simulink model "ssc_auto_ev_20b"  (R2020b)
settings: Solver=VariableStepAuto  StartTime=0.0  StopTime=200  RelTol=1e-3  AbsTol=1e-3
PreLoadFcn:
  | % Simulation parameters
  | dt = 0.01;
  | 
  | % Battery cell parameters
  | ssc_lithium_cell_1RC_ini
  | Nseries = 100;
  | Nparallel = 10;
  | 
  | % Motor parameters
  | max_torque = 220;
  | max_power = 80e3;
  | 
  | % Vehicle parameters
  | vehicle_mass = 4000;
  | wheel_radius = 0.35;
  | area = 5;
  | drag_coefficient = 0.25;
  | air_density = 1.225;
  | gravity = 9.81;
  | rolling_res_ratio = 0.015;
  | 
  | % Differential drive parameters
  | gear_ratio = 12;
  | 
  | % Simplified braking system parameters
  | force_max_pedal = 500;
  | braking_torque_to_pedal_force_ratio = -16;
  | 
  | % Vehicle controller parameters
  | hill_hold_max_speed = 0.5;
  | 
  | % Water properties for cooling circuit
  | load WaterProperties
  | 
  | % Input signals for Signal Editor block
  | load ssc_auto_ev_Inputs
values from neighbouring files (symbols this model uses):
  C1_LUT = [1913.6 4625.7 23306 10736 18036 12251 9022.9 12447 18872 40764 18721 33630 ... (21 elements, 7x3)]    [ssc_auto_ev_param.mat]
  Capacity_LUT = [28.0081 27.625 27.6392]    [ssc_auto_ev_param.mat]
  cell_Cp_heat = 810.5328    [ssc_auto_ev_param.mat]
  cell_mass = 1    [ssc_auto_ev_param.mat]
  Em_LUT = [3.4966 3.5519 3.6183 3.7066 3.9131 4.0748 4.1923 3.5057 3.566 3.6337 3.7127 3.9259 ... (21 elements, 7x3)]    [ssc_auto_ev_param.mat]
  Qe_init = 15.6845    [ssc_auto_ev_param.mat]
  R0_LUT = [0.0117 0.011 0.0114 0.0107 0.0107 0.0113 0.0116 0.0085 0.0085 0.0087 0.0082 0.0083 ... (21 elements, 7x3)]    [ssc_auto_ev_param.mat]
  R1_LUT = [0.0109 0.0069 0.0047 0.0034 0.0033 0.0033 0.0028 0.0029 0.0024 0.0026 0.0016 0.0023 ... (21 elements, 7x3)]    [ssc_auto_ev_param.mat]
  SOC_LUT = [0 0.1 0.25 0.5 0.75 0.9 1]    [ssc_auto_ev_param.mat]
  T_init = 293.15    [ssc_auto_ev_param.mat]
  Temperature_LUT = [278.15 293.15 313.15]    [ssc_auto_ev_param.mat]
undefined symbols (not defined in the file or in its folder): DiscIntNeverNeededParam, K, Lambda, tau, x0
libraries: fl_lib x656, nesl_utility x86, simulink x21, LiBatteryElements_lib x16, SignalEditorBlockLib x4, simulink_extras x4
(part 6 of 13)

== system ssc_auto_ev_20b/Step 3: Ungroup and Redraw/Motor Drive ==
  iRef : Inport
  DC Motor1 : Subsystem  Tag=PublishSubsystem
      mask Display:
      | % Circle, in/out, and 'M'
      | image('ssc_dcmotor_maskicon.png');
      | 
      | % % Circle
      | % plot(sin(0:0.1:2.2*pi)*0.9,cos(0:0.1:2.2*pi)*0.9);
      | %
      | % % In/out
      | % plot([-1.3 -0.9],[0 0]);
      | % plot([1.3 0.9],[0 0]);
      | %
      | % % 'M'
      | % plot([0.5 0.5],[-0.5 0.5]);
      | % plot([-0.5 -0.5],[-0.5 0.5]);
      | % plot([0.5 0],[0.5 -0.5]);
      | % plot([-0.5 0],[0.5 -0.5]);
      | 
      | % Plot points to set plot range
      | color('white');plot(1.5,1.5);plot(-1.5,-1.5)
      | color('black');
      | 
      | port_label('RConn',1,'R');
      | port_label('RConn',2,'C');
      | port_label('LConn',1,'V+');
      | port_label('LConn',2,'V-');
  DC Motor2 : Subsystem  Tag=PublishSubsystem
      mask Display:
      | % Circle, in/out, and 'M'
      | image('ssc_dcmotor_maskicon.png');
      | 
      | % % Circle
      | % plot(sin(0:0.1:2.2*pi)*0.9,cos(0:0.1:2.2*pi)*0.9);
      | %
      | % % In/out
      | % plot([-1.3 -0.9],[0 0]);
      | % plot([1.3 0.9],[0 0]);
      | %
      | % % 'M'
      | % plot([0.5 0.5],[-0.5 0.5]);
      | % plot([-0.5 -0.5],[-0.5 0.5]);
      | % plot([0.5 0],[0.5 -0.5]);
      | % plot([-0.5 0],[0.5 -0.5]);
      | 
      | % Plot points to set plot range
      | color('white');plot(1.5,1.5);plot(-1.5,-1.5)
      | color('black');
      | 
      | port_label('RConn',1,'R');
      | port_label('RConn',2,'C');
      | port_label('LConn',1,'V+');
      | port_label('LConn',2,'V-');
  Ideal Rotational Motion Sensor : fl_lib/Mechanical/Mechanical Sensors/Ideal Rotational Motion Sensor  wrap_angle=simscape.enum.onoff.off  offset=0 rad
      settings: SourceProductBaseCode=PW,SS,VE
  MRRef : fl_lib/Mechanical/Rotational Elements/Mechanical Rotational Reference
      settings: SourceProductBaseCode=PW,SS,VE
  MRRef1 : fl_lib/Mechanical/Rotational Elements/Mechanical Rotational Reference
      settings: SourceProductBaseCode=PW,SS,VE
  MRRef2 : fl_lib/Mechanical/Rotational Elements/Mechanical Rotational Reference
      settings: SourceProductBaseCode=PW,SS,VE
  Motor Torque Controller 1 (System-Level Representation) : Subsystem
      settings: PortSchema="{\"entries\":[{\"content\":{\"sides\":[{\"content\":{\"connectorIds\":[\"LConn1\",\"LConn2\"]},\"type\":\"ConnectorPlacement.EquallySpacedRectSide\",\"uuid\":\"fa610323-4e51-4b68-84d8-5520af174050\"},{\"content\":{\"connectorIds\":[\"RConn1\",\"RConn2\"],\"side\":\"RIGHT\"},\"type\":\"ConnectorPlacement.EquallySpacedRectSide\",\"uuid\":\"4363b90b-a4e0-4b49-9dec-cc6d130d9345\"},{\"content\":{\"connectorIds\":[\"LConn3\"],\"side\":\"TOP\"},\"type\":\"ConnectorPlacement.EquallySpacedRectSide\",\"uuid\":\"1b5285b6-bf42-4633-bccd-78a8c0464c36\"}]},\"type\":\"ConnectorPlacement.EquallySpacedConnector\",\"uuid\":\"5522e717-4ae9-420d-ac3d-a671d244aac1\"}],\"packageUris\":[\"http://schema.mathworks.com/mf0/Connector/R2020b\"],\"version\":\"1.0\"}"
  Motor Torque Controller 1 (System-Level Representation)1 : Subsystem
      settings: PortSchema="{\"entries\":[{\"content\":{\"sides\":[{\"content\":{\"connectorIds\":[\"LConn1\",\"LConn2\"]},\"type\":\"ConnectorPlacement.EquallySpacedRectSide\",\"uuid\":\"fa610323-4e51-4b68-84d8-5520af174050\"},{\"content\":{\"connectorIds\":[\"RConn1\",\"RConn2\"],\"side\":\"RIGHT\"},\"type\":\"ConnectorPlacement.EquallySpacedRectSide\",\"uuid\":\"4363b90b-a4e0-4b49-9dec-cc6d130d9345\"},{\"content\":{\"connectorIds\":[\"LConn3\"],\"side\":\"TOP\"},\"type\":\"ConnectorPlacement.EquallySpacedRectSide\",\"uuid\":\"1b5285b6-bf42-4633-bccd-78a8c0464c36\"}]},\"type\":\"ConnectorPlacement.EquallySpacedConnector\",\"uuid\":\"5522e717-4ae9-420d-ac3d-a671d244aac1\"}],\"packageUris\":[\"http://schema.mathworks.com/mf0/Connector/R2020b\"],\"version\":\"1.0\"}"
  Sensing wMotor : Subsystem
      mask Display: disp('w');
  Simulink-PS G1 : nesl_utility/Simulink-PS Converter  PhysicalDomain=network_engine_domain  SubClassName=ps_input  LeftPortType=input  RightPortType=output  PseudoPeriodic=off  Frequencies=[]  NoiseDistribution=none  NoiseParameters=[]  Unit=A  AffineConversion=off  FilteringAndDerivatives=zero  SimscapeFilterOrder=1  InputFilterTimeConstant=1e-6  UdotUserProvided=1
      settings: SourceProductBaseCode=SS,PW,VE
  Winding-Iron Conductance/1 : fl_lib/Thermal/Thermal Elements/Conductive Heat Transfer  area=250 cm^2  thickness=0.2 cm  th_cond=360 W/(m*K)  T_specify=off  T_priority=None  T=0 K  T_nominal_specify=off  T_nominal_unit=K  T_nominal_value=1  Q_specify=off  Q_priority=None  Q=0 W  Q_nominal_specify=off  Q_nominal_unit=W  Q_nominal_value=1
      settings: SourceProductBaseCode=PW,SS,VE
  Winding-Iron Conductance/2 : fl_lib/Thermal/Thermal Elements/Conductive Heat Transfer  area=250 cm^2  thickness=0.2 cm  th_cond=360 W/(m*K)  T_specify=off  T_priority=None  T=0 K  T_nominal_specify=off  T_nominal_unit=K  T_nominal_value=1  Q_specify=off  Q_priority=None  Q=0 W  Q_nominal_specify=off  Q_nominal_unit=W  Q_nominal_value=1
      settings: SourceProductBaseCode=PW,SS,VE
  + : PMIOPort  Side=Left
  - : PMIOPort  Port=2  Side=Left
  R : PMIOPort  Port=3  Side=Right
  M1 : PMIOPort  Port=4  Side=Left
  M2 : PMIOPort  Port=5  Side=Left
  w : Outport  VectorParamsAs1DForOutWhenUnconnected=off
  wires:
  iRef/1 -> Simulink-PS G1/1
  Sensing wMotor/1(SL) -> w/1
  connections:
  M2/RConn1 -- Winding-Iron Conductance/2/LConn1
  M1/RConn1 -- Winding-Iron Conductance/1/LConn1
  Winding-Iron Conductance/2/RConn1 -- DC Motor2/LConn3
  Winding-Iron Conductance/1/RConn1 -- DC Motor1/LConn3
  DC Motor2/LConn2 -- Motor Torque Controller 1 (System-Level Representation)1/LConn2
  DC Motor2/LConn1 -- Motor Torque Controller 1 (System-Level Representation)1/LConn1
  DC Motor2/RConn2 -- MRRef2/LConn1
  Motor Torque Controller 1 (System-Level Representation)1/LConn3 -- Motor Torque Controller 1 (System-Level Representation)/LConn3 -- Simulink-PS G1/RConn1
  DC Motor1/LConn2 -- Motor Torque Controller 1 (System-Level Representation)/LConn2
  Motor Torque Controller 1 (System-Level Representation)/RConn2 -- Motor Torque Controller 1 (System-Level Representation)1/RConn2 -- -/RConn1
  Motor Torque Controller 1 (System-Level Representation)/RConn1 -- Motor Torque Controller 1 (System-Level Representation)1/RConn1 -- +/RConn1
  Motor Torque Controller 1 (System-Level Representation)/LConn1 -- DC Motor1/LConn1
  MRRef1/LConn1 -- Ideal Rotational Motion Sensor/RConn1
  DC Motor1/RConn2 -- MRRef/LConn1
  R/RConn1 -- Ideal Rotational Motion Sensor/LConn1 -- DC Motor2/RConn1 -- DC Motor1/RConn1
  Ideal Rotational Motion Sensor/RConn2 -- Sensing wMotor/LConn1

== system ssc_auto_ev_20b/Step 3: Ungroup and Redraw/Port 1 Interface ==
  heat flow : Inport
  Controlled Temperature Source : fl_lib/Thermal/Thermal Sources/Controlled Temperature Source
      settings: SourceProductBaseCode=PW,SS,VE
  Heat Flow Rate Sensor : fl_lib/Thermal/Thermal Sensors/Heat Flow Rate Sensor
      settings: SourceProductBaseCode=PW,SS,VE
  Interface : Subsystem  Variant=on  VariantControlMode=label  VariantControl=Variant1  LabelModeActiveChoice=Discrete
      settings: PortSchema="{\"entries\":[{\"content\":{\"sides\":[{\"content\":{\"connectorIds\":[\"In1\",\"Out2\"]},\"type\":\"ConnectorPlacement.EquallySpacedRectSide\",\"uuid\":\"aa56821c-7799-44e3-b228-553c5b43a68d\"},{\"content\":{\"connectorIds\":[\"In2\",\"Out1\"],\"side\":\"RIGHT\"},\"type\":\"ConnectorPlacement.EquallySpacedRectSide\",\"uuid\":\"8658dee5-55e2-4f33-bdec-e6600ce27fc1\"},{\"content\":{\"connectorIds\":[],\"side\":\"TOP\"},\"type\":\"ConnectorPlacement.EquallySpacedRectSide\",\"uuid\":\"2effe9c6-8e61-4f0c-a39b-329d9ffc707d\"}]},\"type\":\"ConnectorPlacement.EquallySpacedConnector\",\"uuid\":\"c8fc8444-dfc7-49a5-9550-b957635f7d8f\"}],\"packageUris\":[\"http://schema.mathworks.com/mf0/Connector/R2020b\"],\"version\":\"1.0\"}"
  T1 : nesl_utility/Simulink-PS Converter  PhysicalDomain=network_engine_domain  SubClassName=ps_input  LeftPortType=input  RightPortType=output  PseudoPeriodic=off  Frequencies=[]  NoiseDistribution=none  NoiseParameters=[]  Unit=K  AffineConversion=off  FilteringAndDerivatives=provide  SimscapeFilterOrder=1  InputFilterTimeConstant=0.001  UdotUserProvided=0
      settings: SourceProductBaseCode=SS,PW,VE
  Thermal Reference : fl_lib/Thermal/Thermal Elements/Thermal Reference
      settings: SourceProductBaseCode=PW,SS,VE
  q1 : nesl_utility/PS-Simulink Converter  PhysicalDomain=network_engine_domain  SubClassName=ps_output  LeftPortType=input  RightPortType=output  PseudoPeriodic=off  Frequencies=[]  Unit=W  AffineConversion=off
      settings: SourceProductBaseCode=SS,PW,VE
  1 : PMIOPort  Side=Left
  temperature : Outport
  wires:
  Interface/1(across2) -> temperature/1
  q1/1 -> Interface/1(through1)
  heat flow/1 -> Interface/2(through2)
  Interface/2(across1) -> T1/1
  connections:
  Heat Flow Rate Sensor/RConn2 -- Controlled Temperature Source/LConn1
  Heat Flow Rate Sensor/LConn1 -- 1/RConn1
  q1/LConn1 -- Heat Flow Rate Sensor/RConn1
  Thermal Reference/LConn1 -- Controlled Temperature Source/RConn2
  Controlled Temperature Source/RConn1 -- T1/RConn1

== system ssc_auto_ev_20b/Step 3: Ungroup and Redraw/Port 1 Interface1 ==
  heat flow : Inport
  Controlled Temperature Source : fl_lib/Thermal/Thermal Sources/Controlled Temperature Source
      settings: SourceProductBaseCode=PW,SS,VE
  Heat Flow Rate Sensor : fl_lib/Thermal/Thermal Sensors/Heat Flow Rate Sensor
      settings: SourceProductBaseCode=PW,SS,VE
  Interface : Subsystem  Variant=on  VariantControlMode=label  VariantControl=Variant1  LabelModeActiveChoice=Discrete
      settings: PortSchema="{\"entries\":[{\"content\":{\"sides\":[{\"content\":{\"connectorIds\":[\"In1\",\"Out2\"]},\"type\":\"ConnectorPlacement.EquallySpacedRectSide\",\"uuid\":\"aa56821c-7799-44e3-b228-553c5b43a68d\"},{\"content\":{\"connectorIds\":[\"In2\",\"Out1\"],\"side\":\"RIGHT\"},\"type\":\"ConnectorPlacement.EquallySpacedRectSide\",\"uuid\":\"8658dee5-55e2-4f33-bdec-e6600ce27fc1\"},{\"content\":{\"connectorIds\":[],\"side\":\"TOP\"},\"type\":\"ConnectorPlacement.EquallySpacedRectSide\",\"uuid\":\"2effe9c6-8e61-4f0c-a39b-329d9ffc707d\"}]},\"type\":\"ConnectorPlacement.EquallySpacedConnector\",\"uuid\":\"c8fc8444-dfc7-49a5-9550-b957635f7d8f\"}],\"packageUris\":[\"http://schema.mathworks.com/mf0/Connector/R2020b\"],\"version\":\"1.0\"}"
  T1 : nesl_utility/Simulink-PS Converter  PhysicalDomain=network_engine_domain  SubClassName=ps_input  LeftPortType=input  RightPortType=output  PseudoPeriodic=off  Frequencies=[]  NoiseDistribution=none  NoiseParameters=[]  Unit=K  AffineConversion=off  FilteringAndDerivatives=provide  SimscapeFilterOrder=1  InputFilterTimeConstant=0.001  UdotUserProvided=0
      settings: SourceProductBaseCode=SS,PW,VE
  Thermal Reference : fl_lib/Thermal/Thermal Elements/Thermal Reference
      settings: SourceProductBaseCode=PW,SS,VE
  q1 : nesl_utility/PS-Simulink Converter  PhysicalDomain=network_engine_domain  SubClassName=ps_output  LeftPortType=input  RightPortType=output  PseudoPeriodic=off  Frequencies=[]  Unit=W  AffineConversion=off
      settings: SourceProductBaseCode=SS,PW,VE
  1 : PMIOPort  Side=Left
  temperature : Outport
  wires:
  Interface/1(across2) -> temperature/1
  q1/1 -> Interface/1(through1)
  heat flow/1 -> Interface/2(through2)
  Interface/2(across1) -> T1/1
  connections:
  Heat Flow Rate Sensor/RConn2 -- Controlled Temperature Source/LConn1
  Heat Flow Rate Sensor/LConn1 -- 1/RConn1
  q1/LConn1 -- Heat Flow Rate Sensor/RConn1
  Thermal Reference/LConn1 -- Controlled Temperature Source/RConn2
  Controlled Temperature Source/RConn1 -- T1/RConn1

== system ssc_auto_ev_20b/Step 3: Ungroup and Redraw/Port 1 Interface2 ==
  heat flow : Inport
  Controlled Temperature Source : fl_lib/Thermal/Thermal Sources/Controlled Temperature Source
      settings: SourceProductBaseCode=PW,SS,VE
  Heat Flow Rate Sensor : fl_lib/Thermal/Thermal Sensors/Heat Flow Rate Sensor
      settings: SourceProductBaseCode=PW,SS,VE
  Interface : Subsystem  Variant=on  VariantControlMode=label  VariantControl=Variant1  LabelModeActiveChoice=Discrete
      settings: PortSchema="{\"entries\":[{\"content\":{\"sides\":[{\"content\":{\"connectorIds\":[\"In1\",\"Out2\"]},\"type\":\"ConnectorPlacement.EquallySpacedRectSide\",\"uuid\":\"aa56821c-7799-44e3-b228-553c5b43a68d\"},{\"content\":{\"connectorIds\":[\"In2\",\"Out1\"],\"side\":\"RIGHT\"},\"type\":\"ConnectorPlacement.EquallySpacedRectSide\",\"uuid\":\"8658dee5-55e2-4f33-bdec-e6600ce27fc1\"},{\"content\":{\"connectorIds\":[],\"side\":\"TOP\"},\"type\":\"ConnectorPlacement.EquallySpacedRectSide\",\"uuid\":\"2effe9c6-8e61-4f0c-a39b-329d9ffc707d\"}]},\"type\":\"ConnectorPlacement.EquallySpacedConnector\",\"uuid\":\"c8fc8444-dfc7-49a5-9550-b957635f7d8f\"}],\"packageUris\":[\"http://schema.mathworks.com/mf0/Connector/R2020b\"],\"version\":\"1.0\"}"
  T1 : nesl_utility/Simulink-PS Converter  PhysicalDomain=network_engine_domain  SubClassName=ps_input  LeftPortType=input  RightPortType=output  PseudoPeriodic=off  Frequencies=[]  NoiseDistribution=none  NoiseParameters=[]  Unit=K  AffineConversion=off  FilteringAndDerivatives=provide  SimscapeFilterOrder=1  InputFilterTimeConstant=0.001  UdotUserProvided=0
      settings: SourceProductBaseCode=SS,PW,VE
  Thermal Reference : fl_lib/Thermal/Thermal Elements/Thermal Reference
      settings: SourceProductBaseCode=PW,SS,VE
  q1 : nesl_utility/PS-Simulink Converter  PhysicalDomain=network_engine_domain  SubClassName=ps_output  LeftPortType=input  RightPortType=output  PseudoPeriodic=off  Frequencies=[]  Unit=W  AffineConversion=off
      settings: SourceProductBaseCode=SS,PW,VE
  1 : PMIOPort  Side=Left
  temperature : Outport
  wires:
  Interface/2(across1) -> T1/1
  heat flow/1 -> Interface/2(through2)
  q1/1 -> Interface/1(through1)
  Interface/1(across2) -> temperature/1
  connections:
  Controlled Temperature Source/RConn1 -- T1/RConn1
  Thermal Reference/LConn1 -- Controlled Temperature Source/RConn2
  q1/LConn1 -- Heat Flow Rate Sensor/RConn1
  Heat Flow Rate Sensor/LConn1 -- 1/RConn1
  Heat Flow Rate Sensor/RConn2 -- Controlled Temperature Source/LConn1

== system ssc_auto_ev_20b/Step 3: Ungroup and Redraw/Port 1 Interface3 ==
  voltage : Inport
  Controlled Voltage Source : fl_lib/Electrical/Electrical Sources/Controlled Voltage Source
      settings: SourceProductBaseCode=PW,SS,VE
  Current Sensor : fl_lib/Electrical/Electrical Sensors/Current Sensor
      settings: SourceProductBaseCode=PW,SS,VE
  Electrical Reference : fl_lib/Electrical/Electrical Elements/Electrical Reference
      settings: SourceProductBaseCode=PW,SS,VE
  Interface : Subsystem  Variant=on  VariantControlMode=label  VariantControl=Variant1  LabelModeActiveChoice=Discrete
      settings: PortSchema="{\"entries\":[{\"content\":{\"sides\":[{\"content\":{\"connectorIds\":[\"In1\",\"Out2\"]},\"type\":\"ConnectorPlacement.EquallySpacedRectSide\",\"uuid\":\"aa56821c-7799-44e3-b228-553c5b43a68d\"},{\"content\":{\"connectorIds\":[\"In2\",\"Out1\"],\"side\":\"RIGHT\"},\"type\":\"ConnectorPlacement.EquallySpacedRectSide\",\"uuid\":\"8658dee5-55e2-4f33-bdec-e6600ce27fc1\"},{\"content\":{\"connectorIds\":[],\"side\":\"TOP\"},\"type\":\"ConnectorPlacement.EquallySpacedRectSide\",\"uuid\":\"2effe9c6-8e61-4f0c-a39b-329d9ffc707d\"}]},\"type\":\"ConnectorPlacement.EquallySpacedConnector\",\"uuid\":\"c8fc8444-dfc7-49a5-9550-b957635f7d8f\"}],\"packageUris\":[\"http://schema.mathworks.com/mf0/Connector/R2020b\"],\"version\":\"1.0\"}"
  Ip : nesl_utility/PS-Simulink Converter  PhysicalDomain=network_engine_domain  SubClassName=ps_output  LeftPortType=input  RightPortType=output  PseudoPeriodic=off  Frequencies=[]  Unit=A  AffineConversion=off
      settings: SourceProductBaseCode=SS,PW,VE
  Vp : nesl_utility/Simulink-PS Converter  PhysicalDomain=network_engine_domain  SubClassName=ps_input  LeftPortType=input  RightPortType=output  PseudoPeriodic=off  Frequencies=[]  NoiseDistribution=none  NoiseParameters=[]  Unit=V  AffineConversion=off  FilteringAndDerivatives=zero  SimscapeFilterOrder=1  InputFilterTimeConstant=0.001  UdotUserProvided=1
      settings: SourceProductBaseCode=SS,PW,VE
  1 : PMIOPort  Side=Left
  current : Outport
  wires:
  voltage/1 -> Interface/2(across2)
  Interface/2(across1) -> Vp/1
  Ip/1 -> Interface/1(through1)
  Interface/1(through2) -> current/1
  connections:
  Vp/RConn1 -- Controlled Voltage Source/RConn1
  1/RConn1 -- Current Sensor/LConn1
  Current Sensor/RConn2 -- Controlled Voltage Source/LConn1
  Current Sensor/RConn1 -- Ip/LConn1
  Electrical Reference/LConn1 -- Controlled Voltage Source/RConn2

== system ssc_auto_ev_20b/Step 3: Ungroup and Redraw/Port 2 Interface ==
  temperature : Inport
  Controlled Temperature Source : fl_lib/Thermal/Thermal Sources/Controlled Temperature Source
      settings: SourceProductBaseCode=PW,SS,VE
  Heat Flow Rate Sensor : fl_lib/Thermal/Thermal Sensors/Heat Flow Rate Sensor
      settings: SourceProductBaseCode=PW,SS,VE
  T2 : nesl_utility/Simulink-PS Converter  PhysicalDomain=network_engine_domain  SubClassName=ps_input  LeftPortType=input  RightPortType=output  PseudoPeriodic=off  Frequencies=[]  NoiseDistribution=none  NoiseParameters=[]  Unit=K  AffineConversion=off  FilteringAndDerivatives=provide  SimscapeFilterOrder=1  InputFilterTimeConstant=0.001  UdotUserProvided=0
      settings: SourceProductBaseCode=SS,PW,VE
  Thermal Reference : fl_lib/Thermal/Thermal Elements/Thermal Reference
      settings: SourceProductBaseCode=PW,SS,VE
  q2 : nesl_utility/PS-Simulink Converter  PhysicalDomain=network_engine_domain  SubClassName=ps_output  LeftPortType=input  RightPortType=output  PseudoPeriodic=off  Frequencies=[]  Unit=W  AffineConversion=off
      settings: SourceProductBaseCode=SS,PW,VE
  2 : PMIOPort  Side=Right
  heat flow : Outport
  wires:
  q2/1 -> heat flow/1
  temperature/1 -> T2/1
  connections:
  Heat Flow Rate Sensor/RConn2 -- Controlled Temperature Source/LConn1
  Thermal Reference/LConn1 -- Controlled Temperature Source/RConn2
  Heat Flow Rate Sensor/LConn1 -- 2/RConn1
  T2/RConn1 -- Controlled Temperature Source/RConn1
  q2/LConn1 -- Heat Flow Rate Sensor/RConn1

== system ssc_auto_ev_20b/Step 3: Ungroup and Redraw/Port 2 Interface1 ==
  temperature : Inport
  Controlled Temperature Source : fl_lib/Thermal/Thermal Sources/Controlled Temperature Source
      settings: SourceProductBaseCode=PW,SS,VE
  Heat Flow Rate Sensor : fl_lib/Thermal/Thermal Sensors/Heat Flow Rate Sensor
      settings: SourceProductBaseCode=PW,SS,VE
  T2 : nesl_utility/Simulink-PS Converter  PhysicalDomain=network_engine_domain  SubClassName=ps_input  LeftPortType=input  RightPortType=output  PseudoPeriodic=off  Frequencies=[]  NoiseDistribution=none  NoiseParameters=[]  Unit=K  AffineConversion=off  FilteringAndDerivatives=provide  SimscapeFilterOrder=1  InputFilterTimeConstant=0.001  UdotUserProvided=0
      settings: SourceProductBaseCode=SS,PW,VE
  Thermal Reference : fl_lib/Thermal/Thermal Elements/Thermal Reference
      settings: SourceProductBaseCode=PW,SS,VE
  q2 : nesl_utility/PS-Simulink Converter  PhysicalDomain=network_engine_domain  SubClassName=ps_output  LeftPortType=input  RightPortType=output  PseudoPeriodic=off  Frequencies=[]  Unit=W  AffineConversion=off
      settings: SourceProductBaseCode=SS,PW,VE
  2 : PMIOPort  Side=Right
  heat flow : Outport
  wires:
  q2/1 -> heat flow/1
  temperature/1 -> T2/1
  connections:
  Heat Flow Rate Sensor/RConn2 -- Controlled Temperature Source/LConn1
  Thermal Reference/LConn1 -- Controlled Temperature Source/RConn2
  Heat Flow Rate Sensor/LConn1 -- 2/RConn1
  T2/RConn1 -- Controlled Temperature Source/RConn1
  q2/LConn1 -- Heat Flow Rate Sensor/RConn1

== system ssc_auto_ev_20b/Step 3: Ungroup and Redraw/Port 2 Interface2 ==
  temperature : Inport
  Controlled Temperature Source : fl_lib/Thermal/Thermal Sources/Controlled Temperature Source
      settings: SourceProductBaseCode=PW,SS,VE
  Heat Flow Rate Sensor : fl_lib/Thermal/Thermal Sensors/Heat Flow Rate Sensor
      settings: SourceProductBaseCode=PW,SS,VE
  T2 : nesl_utility/Simulink-PS Converter  PhysicalDomain=network_engine_domain  SubClassName=ps_input  LeftPortType=input  RightPortType=output  PseudoPeriodic=off  Frequencies=[]  NoiseDistribution=none  NoiseParameters=[]  Unit=K  AffineConversion=off  FilteringAndDerivatives=provide  SimscapeFilterOrder=1  InputFilterTimeConstant=0.001  UdotUserProvided=0
      settings: SourceProductBaseCode=SS,PW,VE
  Thermal Reference : fl_lib/Thermal/Thermal Elements/Thermal Reference
      settings: SourceProductBaseCode=PW,SS,VE
  q2 : nesl_utility/PS-Simulink Converter  PhysicalDomain=network_engine_domain  SubClassName=ps_output  LeftPortType=input  RightPortType=output  PseudoPeriodic=off  Frequencies=[]  Unit=W  AffineConversion=off
      settings: SourceProductBaseCode=SS,PW,VE
  2 : PMIOPort  Side=Right
  heat flow : Outport
  wires:
  temperature/1 -> T2/1
  q2/1 -> heat flow/1
  connections:
  q2/LConn1 -- Heat Flow Rate Sensor/RConn1
  T2/RConn1 -- Controlled Temperature Source/RConn1
  Heat Flow Rate Sensor/LConn1 -- 2/RConn1
  Thermal Reference/LConn1 -- Controlled Temperature Source/RConn2
  Heat Flow Rate Sensor/RConn2 -- Controlled Temperature Source/LConn1

== system ssc_auto_ev_20b/Step 3: Ungroup and Redraw/Port 2 Interface3 ==
  current : Inport
  Controlled Current Source : fl_lib/Electrical/Electrical Sources/Controlled Current Source
      settings: SourceProductBaseCode=PW,SS,VE
  Electrical Reference : fl_lib/Electrical/Electrical Elements/Electrical Reference
      settings: SourceProductBaseCode=PW,SS,VE
  Electrical Reference1 : fl_lib/Electrical/Electrical Elements/Electrical Reference
      settings: SourceProductBaseCode=PW,SS,VE
  In : nesl_utility/Simulink-PS Converter  PhysicalDomain=network_engine_domain  SubClassName=ps_input  LeftPortType=input  RightPortType=output  PseudoPeriodic=off  Frequencies=[]  NoiseDistribution=none  NoiseParameters=[]  Unit=A  AffineConversion=off  FilteringAndDerivatives=zero  SimscapeFilterOrder=1  InputFilterTimeConstant=0.001  UdotUserProvided=1
      settings: SourceProductBaseCode=SS,PW,VE
  Vn : nesl_utility/PS-Simulink Converter  PhysicalDomain=network_engine_domain  SubClassName=ps_output  LeftPortType=input  RightPortType=output  PseudoPeriodic=off  Frequencies=[]  Unit=V  AffineConversion=off
      settings: SourceProductBaseCode=SS,PW,VE
  Voltage Sensor : fl_lib/Electrical/Electrical Sensors/Voltage Sensor
      settings: SourceProductBaseCode=PW,SS,VE
  2 : PMIOPort  Side=Right
  voltage : Outport
  wires:
  current/1 -> In/1
  Vn/1 -> voltage/1
  connections:
  In/RConn1 -- Controlled Current Source/RConn1
  Controlled Current Source/LConn1 -- Electrical Reference/LConn1
  Voltage Sensor/RConn1 -- Vn/LConn1
  2/RConn1 -- Controlled Current Source/RConn2 -- Voltage Sensor/LConn1
  Electrical Reference1/LConn1 -- Voltage Sensor/RConn2

== system ssc_auto_ev_20b/Step 3: Ungroup and Redraw/Vehicle Dynamics ==
  Test data : Inport
  Brake Torque : Subsystem
  Bus Selector : BusSelector  OutputSignals=Incline,Wind speed,Brake pedal
  Drag and Gravity : Subsystem
  Final Drive Ratio : fl_lib/Mechanical/Mechanisms/Gear Box  ratio=gear_ratio  t_in_specify=off  t_in_priority=High  t_in=0 N*m  t_in_nominal_specify=off  t_in_nominal_unit=N*m  t_in_nominal_value=1  t_out_specify=off  t_out_priority=High  t_out=0 N*m  t_out_nominal_specify=off  t_out_nominal_unit=N*m  t_out_nominal_value=1
      settings: SourceProductBaseCode=PW,SS,VE
  Force Source : fl_lib/Mechanical/Mechanical Sources/Ideal Force Source
      settings: SourceProductBaseCode=PW,SS,VE
  MTRef : fl_lib/Mechanical/Translational Elements/Mechanical Translational Reference
      settings: SourceProductBaseCode=PW,SS,VE
  PS Subtract : fl_lib/Physical Signals/Functions/PS Subtract
      settings: SourceProductBaseCode=PW,SS,VE
  Sensing Speed : Subsystem
      mask Display: disp('v')
  Vehicle Mass : fl_lib/Mechanical/Translational Elements/Mass  mass=vehicle_mass kg  num_ports=foundation.enum.numPorts2.one  v_specify=off  v_priority=High  v=0 m/s  v_nominal_specify=off  v_nominal_unit=m/s  v_nominal_value=1  f_specify=off  f_priority=High  f=0 N  f_nominal_specify=off  f_nominal_unit=N  f_nominal_value=1
      settings: SourceProductBaseCode=PW,SS,VE
  Wheel and Axle : fl_lib/Mechanical/Mechanisms/Wheel and Axle  R=wheel_radius m  or=1  t_specify=off  t_priority=High  t=0 N*m  t_nominal_specify=off  t_nominal_unit=N*m  t_nominal_value=1  f_specify=off  f_priority=High  f=0 N  f_nominal_specify=off  f_nominal_unit=N  f_nominal_value=1
      settings: SourceProductBaseCode=PW,SS,VE
  R : PMIOPort  Side=Left
  wires:
  Test data/1 -> Bus Selector/1
  Bus Selector/3 -> Brake Torque/1(Pedal)  "<Brake pedal>"
  Bus Selector/1 -> Drag and Gravity/1(beta)  "<Incline>"
  Bus Selector/2 -> Drag and Gravity/2(vW)  "<Wind speed>"
  connections:
  R/RConn1 -- Final Drive Ratio/LConn1
  Force Source/RConn2 -- MTRef/LConn1
  Brake Torque/RConn1 -- Final Drive Ratio/RConn1 -- Wheel and Axle/LConn1
  PS Subtract/RConn1 -- Force Source/RConn1
  Drag and Gravity/LConn3 -- PS Subtract/LConn1
  Drag and Gravity/LConn2 -- PS Subtract/LConn2
  Wheel and Axle/RConn1 -- Sensing Speed/LConn1 -- Force Source/LConn1 -- Vehicle Mass/LConn1
  Drag and Gravity/LConn1 -- Sensing Speed/RConn1

== system ssc_auto_ev_20b/Step 3: Ungroup and Redraw/Vehicle Control ==
  ECU : Inport
  wMeas : Inport  Port=2
  -1 : Gain  Gain=-1
  1/Kt : Gain  Gain=1/1
  Bus Selector : BusSelector  OutputSignals=Cruise enable,Cruise disable,Brake pedal,Throttle,Incline
  Compare To Constant : simulink/Logic and Bit Operations/Compare To Constant  relop=>  const=0  OutDataTypeStr=boolean
  Cruise Control : Subsystem
  Feedforward term for regenerative braking on downhill : Subsystem
  Max Power : Subsystem
  Power limits : simulink/Discontinuities/Saturation Dynamic  OutMin=[]  OutMax=[]  OutDataTypeStr=Inherit: Same as second input  OutDataType=fixdt(1, 16)  OutScaling=2^-10  DoSatur=off
  Switch between torque control and speed control : Switch  Criteria=u2 > Threshold
  Torque limits : Saturate  UpperLimit=max_torque  LowerLimit=-max_torque
  Torque Demand Management : Subsystem
  iRef : Outport  VectorParamsAs1DForOutWhenUnconnected=off
  wires:
  Feedforward term for regenerative braking on downhill/1(Feedfwd trq) -> Torque Demand Management/4(FFbrake)
  1/Kt/1 -> iRef/1
  ECU/1 -> Bus Selector/1
  Cruise Control/2(Enabled) -> Switch between torque control and speed control/2
  Torque Demand Management/1(Dem trq) -> Switch between torque control and speed control/3
  Switch between torque control and speed control/1 -> Torque limits/1
  Bus Selector/1 -> Cruise Control/1(Enable)  "<Cruise enable>"
  wMeas/1 -> Max Power/1(Vspd), Cruise Control/3(wMeas), Torque Demand Management/3(wMeas)
  Cruise Control/1(trqRef) -> Switch between torque control and speed control/1
  Bus Selector/2 -> Cruise Control/2(Disable)  "<Cruise disable>"
  Compare To Constant/1 -> Cruise Control/4(Brake sw)
  Bus Selector/4 -> Torque Demand Management/2(Throttle)  "<Throttle>"
  Bus Selector/3 -> Torque Demand Management/1(Brake), Compare To Constant/1  "<Brake pedal>"
  Bus Selector/5 -> Feedforward term for regenerative braking on downhill/1(Inclin.)  "<Incline>"
  Torque limits/1 -> Power limits/2
  Power limits/1 -> 1/Kt/1
  -1/1 -> Power limits/3
  Max Power/1(Max Power) -> -1/1, Power limits/1

== system ssc_auto_ev_20b/Step 4: Deployment Model/Battery @50Hz ==
  heat flow : Inport
  current : Inport  Port=2
  Battery : Subsystem  mask(Lithium cell (one RC-branch equivalent circuit)){Nseries=Nseries, Nparallel=Nparallel, Qe_init=Qe_init, T_init=T_init, Capacity_LUT=Capacity_LUT, Em_LUT=Em_LUT, R0_LUT=R0_LUT, R1_LUT=R1_LUT, C1_LUT=C1_LUT, cell_mass=cell_mass, cell_Cp_heat=cell_Cp_heat, SOC_LUT=SOC_LUT, Temperature_LUT=Temperature_LUT}
      mask prompts: Nseries "Number of series-connected parallel sets"; Nparallel "Number of parallel-connected cells per parallel set"; Qe_init "Initial cell charge deficit (A*hr)"; T_init "Initial cell temperature (K)"; Capacity_LUT "Capacity (A*hr, 1xN table)"; Em_LUT "Em open-circuit voltage, Em (volts, MxN table)"; R0_LUT "R0 terminal resistance (ohms, MxN table)"; R1_LUT "R1 cell resistance (ohms, MxN table)"; C1_LUT "C1 capacitance (farads, MxN table)"; cell_mass "Cell mass (kg)"; cell_Cp_heat "Cell specific heat (J/kg/K)"; SOC_LUT "SOC table breakpoints (Mx1 array)"; Temperature_LUT "Temperature table breakpoints (K, 1xN array)"
      mask DialogControl ParameterTabVar0 Prompt: Main
      mask DialogControl ParameterTabVar01 Prompt: Electrical (per cell)
      mask DialogControl ParameterTabVar012 Prompt: Thermal (per cell)
      mask DialogControl ParameterTabVar0123 Prompt: Table Breakpoints
      mask Display:
      | % Battery icon
      | plot([1.8 1.3],[0 0])
      | plot([-0.6 -1.6 -1.6 -2.2],[0 0 -0.9 -0.9])
      | patch([1 1 -1 -1]*0.15+0.7,[-1 1 1 -1]*0.4,[0;0;0]);
      | patch([1 1 -1 -1]*0.15-0.6,[-1 1 1 -1]*0.4,[0;0;0]);
      | patch([1 1 -1 -1]*0.15+1.3,[-1 1 1 -1]*0.8,[0;0;0]);
      | patch([1 1 -1 -1]*0.15-0.0,[-1 1 1 -1]*0.8,[0;0;0]);
      | % Thermal port
      | plot([-1.6,-1.3],[1.2,1.2])
      | plot([-1.6,-1.3],[0.5,0.5])
      | plot([-1.6,-2.5],[0.8,0.8])
      | plot(0.2*sin(0:2*pi/50:2*pi)-1.6,0.35*cos(0:2*pi/50:2*pi)+0.85)
      | plot(0.2*sin(0:2*pi/50:pi)-1.3,0.35*cos(0:2*pi/50:pi)+0.85)
      | 
      | % Plot points to set plot range
      | color('white');plot(2.5,1.5);plot(-2.5,-1.5)
  ERef1 : fl_lib/Electrical/Electrical Elements/Electrical Reference
      settings: SourceProductBaseCode=PW,SS,VE
  Port 1 Interface : Subsystem  mask(Network Coupler (Thermal Mass) Port 1 Interface){thermalMass=cell_mass*Nseries*Nparallel*cell_Cp_heat, samplingType=physmod:simscape:couplers:SimscapeNetworkCouplersLib:VariableStepAtPorts1And2_PV, h1=dt*2, h2=dt*5, predictionDiscreteToContinuous=off, smoothingContinuousToDiscrete=off, predictionSlowToFast=off, smoothingFastToSlow=off, nSmooth=1, tsSmoothing=0.01, thermalConductanceNetwork=1, hRecommended=0.001, T0=T_init}
      mask prompts: thermalMass "physmod:simscape:couplers:SimscapeNetworkCouplersLib:ThermalMassJK_MP"; samplingType "physmod:simscape:couplers:SimscapeNetworkCouplersLib:SamplingType_MP"; h1 "physmod:simscape:couplers:SimscapeNetworkCouplersLib:Port1NetworkDiscreteSampleTimes_MP"; h2 "physmod:simscape:couplers:SimscapeNetworkCouplersLib:Port2NetworkDiscreteSampleTimes_MP"; predictionDiscreteToContinuous "physmod:simscape:couplers:SimscapeNetworkCouplersLib:UsePredictionWhenConnectingFixedStepToVariableStep_MP"; smoothingContinuousToDiscrete "physmod:simscape:couplers:SimscapeNetworkCouplersLib:UseSmoothingWhenConnectingVariableStepToFixedStep_MP"; predictionSlowToFast "physmod:simscape:couplers:SimscapeNetworkCouplersLib:UsePredictionWhenConnectingSlowToFastSampleTimes_MP"; smoothingFastToSlow "physmod:simscape:couplers:SimscapeNetworkCouplersLib:UseSmoothingWhenConnectingFastToSlowSampleTimes_MP"; nSmooth "physmod:simscape:couplers:SimscapeNetworkCouplersLib:NumberOfSamplesOverWhichToSmooth_MP"; tsSmoothing "physmod:simscape:couplers:SimscapeNetworkCouplersLib:SmoothingTimeConstants_MP"; thermalConductanceNetwork "physmod:simscape:couplers:SimscapeNetworkCouplersLib:ApproximateConnectedNetworkThermalConductanceWK_MP"; hRecommended "physmod:simscape:couplers:SimscapeNetworkCouplersLib:RecommendedMaxDiscreteSampleTimes_MP"; T0 "physmod:simscape:couplers:SimscapeNetworkCouplersLib:InitialTemperatureK_MP"
      mask help: physmod:simscape:couplers:SimscapeNetworkCouplersLib:NetworkCouplerThermalMassPort1Interface_MD
      mask init: same as ssc_auto_ev_20b/Step 3: Ungroup and Redraw/Port 1 Interface
      settings: PortSchema="{\"entries\":[{\"content\":{\"sides\":[{\"content\":{\"connectorIds\":[\"LConn1\"]},\"type\":\"ConnectorPlacement.EquallySpacedRectSide\",\"uuid\":\"a6d4a9fd-b5aa-40dc-ab7e-2b646b9b57bc\"},{\"content\":{\"connectorIds\":[\"Out1\",\"In1\"],\"side\":\"RIGHT\"},\"type\":\"ConnectorPlacement.EquallySpacedRectSide\",\"uuid\":\"31bb6273-5b9b-48d0-a1a2-6fbacb979b97\"},{\"content\":{\"connectorIds\":[],\"side\":\"TOP\"},\"type\":\"ConnectorPlacement.EquallySpacedRectSide\",\"uuid\":\"0f7afab2-4481-486c-9ad0-2b42c5b091a4\"}]},\"type\":\"ConnectorPlacement.EquallySpacedConnector\",\"uuid\":\"a98e47aa-cbfd-441a-b14c-c9ea515c056e\"}],\"packageUris\":[\"http://schema.mathworks.com/mf0/Connector/R2020b\"],\"version\":\"1.0\"}"
      mask Help: web([docroot '/physmod/simscape/ref/networkcouplerthermalmass.html'])
      mask TypeOptions samplingType: physmod:simscape:couplers:SimscapeNetworkCouplersLib:VariableStepAtPorts1And2_PV | physmod:simscape:couplers:SimscapeNetworkCouplersLib:VariableStepAtPort1AndFixedStepAtPort2_PV | physmod:simscape:couplers:SimscapeNetworkCouplersLib:FixedStepBothPortsWithCommonSampleTime_PV | physmod:simscape:couplers:SimscapeNetworkCouplersLib:FixedStepBothPortsWithFasterSamplingAtPort1_PV
      mask Callback samplingType: foundation.internal.couplers.thermal.parameterVisibilitiesThermalMass(gcb)
      mask Callback predictionDiscreteToContinuous: foundation.internal.couplers.thermal.parameterVisibilitiesThermalMass(gcb)
      mask Callback smoothingContinuousToDiscrete: foundation.internal.couplers.thermal.parameterVisibilitiesThermalMass(gcb)
      mask Callback predictionSlowToFast: foundation.internal.couplers.thermal.parameterVisibilitiesThermalMass(gcb)
      mask Callback smoothingFastToSlow: foundation.internal.couplers.thermal.parameterVisibilitiesThermalMass(gcb)
      mask DialogControl Main Prompt: Main
      mask DialogControl Analysis Prompt: Analysis
      mask DialogControl connectedNetworkInfo Prompt: Connected network information
      mask DialogControl derivedValues Prompt: Derived values
      mask DialogControl updateRecommendations Prompt: Update
      mask DialogControl updateRecommendations Callback: foundation.internal.couplers.thermal.analysisThermalMass(gcb);
      mask DialogControl InitialConditions Prompt: Initial Conditions
  Port 2 Interface3 : Subsystem  mask(Network Coupler (Voltage-Current) Port 2 Interface){}
      mask help: physmod:simscape:couplers:SimscapeNetworkCouplersLib:NetworkCouplerVoltageCurrentPort2Interface_MD
      settings: PortSchema="{\"entries\":[{\"content\":{\"sides\":[{\"content\":{\"connectorIds\":[\"In1\",\"Out1\"]},\"type\":\"ConnectorPlacement.EquallySpacedRectSide\",\"uuid\":\"5a4c1550-e77d-42df-bf3e-b81963920de7\"},{\"content\":{\"connectorIds\":[\"RConn1\"],\"side\":\"RIGHT\"},\"type\":\"ConnectorPlacement.EquallySpacedRectSide\",\"uuid\":\"3fd730f7-5937-4563-a365-595aaae9027b\"},{\"content\":{\"connectorIds\":[],\"side\":\"TOP\"},\"type\":\"ConnectorPlacement.EquallySpacedRectSide\",\"uuid\":\"c16e04e4-26e8-4fd6-98d3-59adbef44c0d\"}]},\"type\":\"ConnectorPlacement.EquallySpacedConnector\",\"uuid\":\"5588d8d0-d459-45fe-a303-1ca6654e99d0\"}],\"packageUris\":[\"http://schema.mathworks.com/mf0/Connector/R2020b\"],\"version\":\"1.0\"}"
      mask Help: web([docroot '/physmod/simscape/ref/networkcouplervoltagecurrent.html'])
  Solver Configuration3 : nesl_utility/Solver Configuration  PhysicalDomain=network_engine_domain  SubClassName=solver  LeftPortType=input  RightPortType=generic  Tones=[]  Harmonics=[]  SimulateNoise=off  Profile=off  UseLocalSampling=off  EnableSwitchedLinearOptims=on  FrequencyDomain=off  UseCCode=off  RelTol=0.001  AbsTol=1e-06  MinStep=1e-09  ToWorkspace=off  RevertToSquareIcSolve=off  NumHomotopyIterations=100  PhasorMode=off  PhasorModeNumHarmonics=1  DoDC=off  ResidualTolerance=1e-9  UseLocalSolver=on  LocalSolverChoice=NE_BACKWARD_EULER_ADVANCER  LocalSolverSampleTime=dt*2  DoFixedCost=on  MaxNonlinIter=3  MaxModeIter=2  ComputeImpulses=off  ImpulseIterations=2  LinearAlgebra=auto  EquationFormulation=NE_TIME_EF  DelaysMemoryBudget=1024  AutomaticFiltering=on  FilteringTimeConstant=0.001  PartitionStorageMethod=AS_NEEDED  PartitionMemoryBudget=1024  PartitionMethod=FAST
      settings: AttributesFormatString=Local Solver: %<UseLocalSolver>  SourceProductBaseCode=SS,PW,VE
  voltage : Outport
  temperature : Outport  Port=2
  wires:
  current/1 -> Port 2 Interface3/1(current)
  heat flow/1 -> Port 1 Interface/1(heat flow)
  Port 1 Interface/1(temperature) -> temperature/1
  Port 2 Interface3/1(voltage) -> voltage/1
  connections:
  Battery/RConn1 -- Port 2 Interface3/RConn1
  ERef1/LConn1 -- Battery/LConn2 -- Solver Configuration3/RConn1
  Battery/LConn1 -- Port 1 Interface/LConn1

== system ssc_auto_ev_20b/Step 4: Deployment Model/Control @100Hz ==
  In1 : Inport
  Driver and Environment : Subsystem
  Unit Delay1 : UnitDelay  SampleTime=dt  HasFrameUpgradeWarning=on
  Vehicle Control : Subsystem  Tag=PublishSubsystem
      settings: PortSchema="{\"entries\":[{\"content\":{\"sides\":[{\"content\":{\"connectorIds\":[\"In1\"]},\"type\":\"ConnectorPlacement.EquallySpacedRectSide\",\"uuid\":\"b68a5c30-2a17-4a0c-a85e-064518f12190\"},{\"content\":{\"connectorIds\":[\"In2\",\"Out1\"],\"side\":\"RIGHT\"},\"type\":\"ConnectorPlacement.EquallySpacedRectSide\",\"uuid\":\"e14e894a-37e1-47c1-8ef8-e46ccf22e5bb\"},{\"content\":{\"connectorIds\":[],\"side\":\"TOP\"},\"type\":\"ConnectorPlacement.EquallySpacedRectSide\",\"uuid\":\"6e722464-54b7-4a5f-a776-dae3a11285e7\"}]},\"type\":\"ConnectorPlacement.EquallySpacedConnector\",\"uuid\":\"82601a10-23cc-4178-a2d7-02b0e1b6e975\"}],\"packageUris\":[\"http://schema.mathworks.com/mf0/Connector/R2020b\"],\"version\":\"1.0\"}"
  ZOH/1 : ZeroOrderHold  SampleTime=dt
  Veh : Outport
  Out2 : Outport  Port=2
  Env : Outport  Port=3
  wires:
  Unit Delay1/1 -> Out2/1
  Vehicle Control/1(iRef) -> Unit Delay1/1
  ZOH/1/1 -> Vehicle Control/2(wMeas)
  Driver and Environment/3(Env) -> Env/1
  Driver and Environment/2(ECU) -> Vehicle Control/1(ECU)
  In1/1 -> ZOH/1/1
  Driver and Environment/1(Veh) -> Veh/1

== system ssc_auto_ev_20b/Step 4: Deployment Model/Thermal @20Hz ==
  T : Inport
  temperature : Inport  Port=2
  temperature1 : Inport  Port=3
  temperature2 : Inport  Port=4
  Cooling System : Subsystem  Tag=PublishSubsystem
      settings: PortSchema="{\"entries\":[{\"content\":{\"sides\":[{\"content\":{\"connectorIds\":[]},\"type\":\"ConnectorPlacement.EquallySpacedRectSide\",\"uuid\":\"d96bbf63-bcbb-4f3a-92bd-eaf78ab4538b\"},{\"content\":{\"connectorIds\":[],\"side\":\"RIGHT\"},\"type\":\"ConnectorPlacement.EquallySpacedRectSide\",\"uuid\":\"b082d3d3-6635-4bf9-9df2-69e4bab78a2b\"},{\"content\":{\"connectorIds\":[\"LConn1\"],\"side\":\"TOP\"},\"type\":\"ConnectorPlacement.EquallySpacedRectSide\",\"uuid\":\"f7177de9-9ba4-478b-b096-87cbc5cd4871\"},{\"content\":{\"connectorIds\":[\"RConn1\"],\"side\":\"BOTTOM\"},\"type\":\"ConnectorPlacement.EquallySpacedRectSide\",\"uuid\":\"4233a269-bfd6-4033-b1ed-0dae7bb50bca\"}]},\"type\":\"ConnectorPlacement.EquallySpacedConnector\",\"uuid\":\"6f10551f-62c9-4564-9ac9-7ef3b87c77d6\"}],\"packageUris\":[\"http://schema.mathworks.com/mf0/Connector/R2020b\"],\"version\":\"1.0\"}"
  Environment : Subsystem
  Motor 1 Thermal Model : Subsystem
  Motor 2 Thermal Model : Subsystem
  Port 2 Interface : Subsystem  mask(Network Coupler (Thermal Mass) Port 2 Interface){}
      mask help: physmod:simscape:couplers:SimscapeNetworkCouplersLib:NetworkCouplerThermalMassPort2Interface_MD
      settings: PortSchema="{\"entries\":[{\"content\":{\"sides\":[{\"content\":{\"connectorIds\":[\"In1\",\"Out1\"]},\"type\":\"ConnectorPlacement.EquallySpacedRectSide\",\"uuid\":\"5a4c1550-e77d-42df-bf3e-b81963920de7\"},{\"content\":{\"connectorIds\":[\"RConn1\"],\"side\":\"RIGHT\"},\"type\":\"ConnectorPlacement.EquallySpacedRectSide\",\"uuid\":\"3fd730f7-5937-4563-a365-595aaae9027b\"},{\"content\":{\"connectorIds\":[],\"side\":\"TOP\"},\"type\":\"ConnectorPlacement.EquallySpacedRectSide\",\"uuid\":\"c16e04e4-26e8-4fd6-98d3-59adbef44c0d\"}]},\"type\":\"ConnectorPlacement.EquallySpacedConnector\",\"uuid\":\"5588d8d0-d459-45fe-a303-1ca6654e99d0\"}],\"packageUris\":[\"http://schema.mathworks.com/mf0/Connector/R2020b\"],\"version\":\"1.0\"}"
      mask Help: web([docroot '/physmod/simscape/ref/networkcouplerthermalmass.html'])
  Port 2 Interface1 : Subsystem  mask(Network Coupler (Thermal Mass) Port 2 Interface){}
      mask help: physmod:simscape:couplers:SimscapeNetworkCouplersLib:NetworkCouplerThermalMassPort2Interface_MD
      settings: PortSchema="{\"entries\":[{\"content\":{\"sides\":[{\"content\":{\"connectorIds\":[\"In1\",\"Out1\"]},\"type\":\"ConnectorPlacement.EquallySpacedRectSide\",\"uuid\":\"5a4c1550-e77d-42df-bf3e-b81963920de7\"},{\"content\":{\"connectorIds\":[\"RConn1\"],\"side\":\"RIGHT\"},\"type\":\"ConnectorPlacement.EquallySpacedRectSide\",\"uuid\":\"3fd730f7-5937-4563-a365-595aaae9027b\"},{\"content\":{\"connectorIds\":[],\"side\":\"TOP\"},\"type\":\"ConnectorPlacement.EquallySpacedRectSide\",\"uuid\":\"c16e04e4-26e8-4fd6-98d3-59adbef44c0d\"}]},\"type\":\"ConnectorPlacement.EquallySpacedConnector\",\"uuid\":\"5588d8d0-d459-45fe-a303-1ca6654e99d0\"}],\"packageUris\":[\"http://schema.mathworks.com/mf0/Connector/R2020b\"],\"version\":\"1.0\"}"
      mask Help: web([docroot '/physmod/simscape/ref/networkcouplerthermalmass.html'])
  Port 2 Interface2 : Subsystem  mask(Network Coupler (Thermal Mass) Port 2 Interface){}
      mask help: physmod:simscape:couplers:SimscapeNetworkCouplersLib:NetworkCouplerThermalMassPort2Interface_MD
      settings: PortSchema="{\"entries\":[{\"content\":{\"sides\":[{\"content\":{\"connectorIds\":[\"In1\",\"Out1\"]},\"type\":\"ConnectorPlacement.EquallySpacedRectSide\",\"uuid\":\"5a4c1550-e77d-42df-bf3e-b81963920de7\"},{\"content\":{\"connectorIds\":[\"RConn1\"],\"side\":\"RIGHT\"},\"type\":\"ConnectorPlacement.EquallySpacedRectSide\",\"uuid\":\"3fd730f7-5937-4563-a365-595aaae9027b\"},{\"content\":{\"connectorIds\":[],\"side\":\"TOP\"},\"type\":\"ConnectorPlacement.EquallySpacedRectSide\",\"uuid\":\"c16e04e4-26e8-4fd6-98d3-59adbef44c0d\"}]},\"type\":\"ConnectorPlacement.EquallySpacedConnector\",\"uuid\":\"5588d8d0-d459-45fe-a303-1ca6654e99d0\"}],\"packageUris\":[\"http://schema.mathworks.com/mf0/Connector/R2020b\"],\"version\":\"1.0\"}"
      mask Help: web([docroot '/physmod/simscape/ref/networkcouplerthermalmass.html'])
  Solver Configuration2 : nesl_utility/Solver Configuration  PhysicalDomain=network_engine_domain  SubClassName=solver  LeftPortType=input  RightPortType=generic  Tones=[]  Harmonics=[]  SimulateNoise=off  Profile=off  UseLocalSampling=off  EnableSwitchedLinearOptims=on  FrequencyDomain=off  UseCCode=off  RelTol=0.001  AbsTol=1e-06  MinStep=1e-09  ToWorkspace=off  RevertToSquareIcSolve=off  NumHomotopyIterations=100  PhasorMode=off  PhasorModeNumHarmonics=1  DoDC=off  ResidualTolerance=1e-9  UseLocalSolver=on  LocalSolverChoice=NE_BACKWARD_EULER_ADVANCER  LocalSolverSampleTime=dt*5  DoFixedCost=on  MaxNonlinIter=3  MaxModeIter=2  ComputeImpulses=off  ImpulseIterations=2  LinearAlgebra=auto  EquationFormulation=NE_TIME_EF  DelaysMemoryBudget=1024  AutomaticFiltering=on  FilteringTimeConstant=0.001  PartitionStorageMethod=AS_NEEDED  PartitionMemoryBudget=1024  PartitionMethod=FAST
      settings: AttributesFormatString=Local Solver: %<UseLocalSolver>  SourceProductBaseCode=SS,PW,VE
  heat flow : Outport
  heat flow1 : Outport  Port=2
  heat flow2 : Outport  Port=3
  wires:
  temperature1/1 -> Port 2 Interface2/1(temperature)
  temperature/1 -> Port 2 Interface/1(temperature)
  Port 2 Interface2/1(heat flow) -> heat flow1/1
  Port 2 Interface/1(heat flow) -> heat flow/1
  T/1 -> Environment/1(T)
  Port 2 Interface1/1(heat flow) -> heat flow2/1
  temperature2/1 -> Port 2 Interface1/1(temperature)
  connections:
  Motor 2 Thermal Model/RConn1 -- Port 2 Interface1/RConn1
  Motor 2 Thermal Model/LConn1 -- Solver Configuration2/RConn1 -- Cooling System/RConn1 -- Environment/RConn1 -- Motor 1 Thermal Model/LConn1
  Motor 1 Thermal Model/RConn1 -- Port 2 Interface2/RConn1
  Cooling System/LConn1 -- Port 2 Interface/RConn1
